simulink model "LQR_Simulation"  (R2022b)
settings: Solver=ode45  StartTime=0.0  StopTime=inf  RelTol=1e-3
values from neighbouring files (symbols this model uses):
  D = 3    [tunningLQR.m]
  xRef = xRef2s    [tunningLQR.m]
  yRef = yRef2s    [tunningLQR.m]
undefined symbols (not defined in the file or in its folder): curvature, esc, hz, path, Q, R_, velocity
libraries: vehdynlibviscommon x1, dspstat3 x1, autolibshared x1
settings Model: Creator=kisho  LastModifiedBy=kisho
settings OptimizationCC: DefaultParameterBehavior=Inlined  EnhancedBackFolding=on  PassReuseOutputArgsAs=Individual arguments  ZeroExternalMemoryAtStartup=off  ZeroInternalMemoryAtStartup=off  MaxStackSize=64  OptimizeBlockOrder=speed  DifferentSizesBufferReuse=on  OptimizationCustomize=off  EfficientTunableParamExpr=on
settings DebuggingCC: ParameterTunabilityLossMsg=error  UnconnectedInputMsg=warning  UnconnectedOutputMsg=warning  UnconnectedLineMsg=warning
settings HardwareCC: ProdBitPerPointer=32  ProdBitPerSizeT=32  ProdBitPerPtrDiffT=32  ProdLargestAtomicFloat=None  ProdIntDivRoundTo=Undefined  ProdEndianess=Unspecified  ProdWordSize=32  ProdHWDeviceType=ASIC/FPGA->ASIC/FPGA  TargetBitPerPointer=64  TargetBitPerSizeT=64  TargetBitPerPtrDiffT=64  TargetLongLongMode=on  TargetIntDivRoundTo=Zero  TargetEndianess=LittleEndian  TargetWordSize=64  TargetHWDeviceType=Custom Processor->MATLAB Host Computer  ProdEqTarget=off
settings ModelReferenceCC: EnableRefExpFcnMdlSchedulingChecks=on
settings SFSimCC: MATLABDynamicMemAlloc=off
settings RTWCC: Description=Embedded Coder  SystemTargetFile=ert.tlc  TemplateMakefile=ert_default_tmf  Toolchain=Catkin  DLArmComputeVersion=19.05
settings CodeAppCC: ForceParamTrailComments=on  IgnoreCustomStorageClasses=off  OperatorAnnotations=on  SimulinkDataObjDesc=on  SFDataObjDesc=on  InsertBlockDesc=on
settings ERTTargetCC: InlinedParameterPlacement=NonHierarchical  ERTCustomFileTemplate=example_file_process.tlc

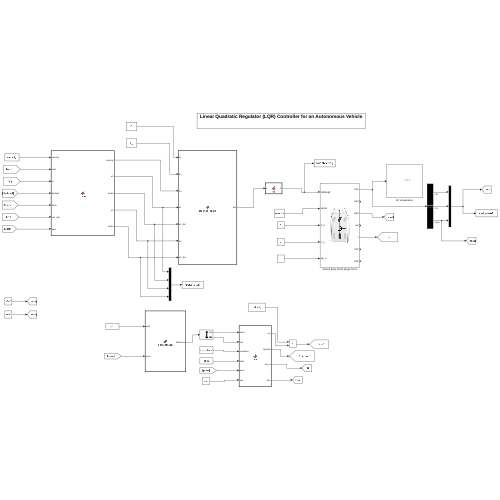
[thumbnail: Simulink's stored preview of the top-level diagram]
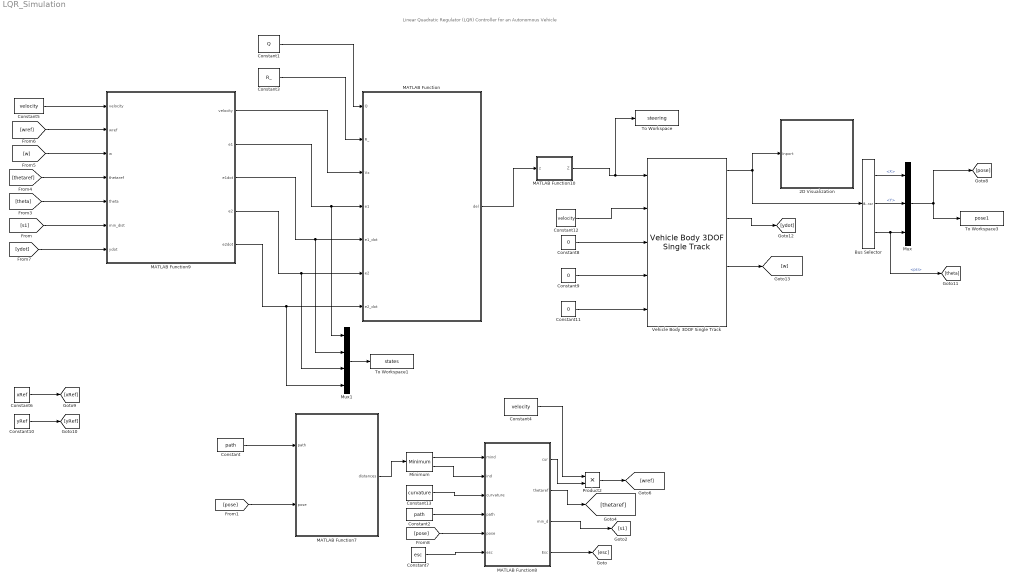
== system LQR_Simulation ==
  note: Linear Quadratic Regulator (LQR) Controller for an Autonomous Vehicle
  2D Visualization : Subsystem
      mask Display: image("visualization.JPG");
  Bus Selector : BusSelector  OutputSignals=InertFrm.Cg.Disp.X,InertFrm.Cg.Disp.Y,InertFrm.Cg.Ang.psi
  Constant : Constant  Value=path  SampleTime=1/hz
  Constant1 : Constant  Value=Q  SampleTime=1/hz
  Constant10 : Constant  Value=yRef  SampleTime=1/hz
  Constant11 : Constant  Value=0  SampleTime=1/hz
  Constant12 : Constant  Value=velocity  SampleTime=1/hz
  Constant13 : Constant  Value=curvature  SampleTime=1/hz
  Constant2 : Constant  Value=path  SampleTime=1/hz
  Constant3 : Constant  Value=R_  SampleTime=1/hz
  Constant4 : Constant  Value=velocity  SampleTime=1/hz
  Constant5 : Constant  Value=velocity  SampleTime=1/hz
  Constant6 : Constant  Value=xRef  SampleTime=1/hz
  Constant7 : Constant  Value=esc  SampleTime=1/hz
  Constant8 : Constant  Value=0  SampleTime=1/hz
  Constant9 : Constant  Value=0  SampleTime=1/hz
  MATLAB Function : MATLAB Function  TreatAsAtomicUnit=on
  MATLAB Function10 : MATLAB Function  TreatAsAtomicUnit=on
  MATLAB Function7 : MATLAB Function  TreatAsAtomicUnit=on
  MATLAB Function8 : MATLAB Function  TreatAsAtomicUnit=on
  MATLAB Function9 : MATLAB Function  TreatAsAtomicUnit=on
  Minimum : dspstat3/Minimum  operation=minimum  fcn=Value and Index  indexBase=One  operateOver=Each row  Dimension=1  InputProcessing=Columns as channels (frame based)  reset=None  roiEnable=off  roiType=Rectangles  roiPortion=Entire ROI  roiOutput=Individual statistics for each ROI  roiFlag=off  roundingMode=Floor  overflowMode=off
  Mux : Mux  Inputs=3
  Mux1 : Mux
  Product2 : Product
  To Workspace : ToWorkspace  VariableName=steering  SaveFormat=Structure With Time  SampleTime=-1
  To Workspace1 : ToWorkspace  VariableName=states  SaveFormat=Structure With Time  SampleTime=-1
  To Workspace3 : ToWorkspace  VariableName=pose1  SaveFormat=Structure With Time  SampleTime=-1
  Vehicle Body 3DOF Single Track : autolibshared/Vehicle Body 3DOF Single Track  trackMode=Single (bicycle)  inputMode=External longitudinal velocity  frontSteerMode=on  rearSteerMode=off  windMode=off  muMode=off  extFMode=off  extMMode=off  htchFMode=off  htchMMode=off  extXo=on  extpsio=on  extxdoto=off  extro=off  extYo=on  extTamb=off  extydoto=off  aMode=2  NF=2  NR=2  m=5  a=0.15  b=0.15  h=0  dh=1  hh=0.2  X_o=0  xdot_o=0  CalphaMode=off  sigmaMode=on  d=0  hl=0  w=[1.4,1.4]  Cy_f=12e3  Cy_r=11e3  sigma_f=.1  sigma_r=.1  alpha_f_brk=[-.1 .1]  Cy_f_data=[-9e3 9e3]  alpha_r_brk=[-.1 .1]  Cy_r_data=[-9e3 9e3]  Y_o=0  ydot_o=0  Izz=0.05  psi_o=0  r_o=0  Af=2  Cd=.3  Cl=.1  Cpm=.1  beta_w=[0 0.01:0.01:0.3]  Cs=[0 0.01:0.01:0.3]  Cym=[0 1e-6:0.01:0.3]  Pabs=101325  Tair=273  g=9.81  mu=1  xdot_tol=.01  Fznom=5000  Fxtire_sat=7e4  Fytire_sat=7e4  longOff=0  latOff=0  vertOff=0  wrapAng=off
  wires:
  MATLAB Function/1(del) -> MATLAB Function10/1(z)
  [s1] -> MATLAB Function9/6(min_dist)
  [theta] -> MATLAB Function9/5(theta)
  [thetaref] -> MATLAB Function9/4(thetaref)
  [w] -> MATLAB Function9/3(w)
  [wref] -> MATLAB Function9/2(wref)
  Constant5/1 -> MATLAB Function9/1("velocity ")
  [ydot] -> MATLAB Function9/7(ydot)
  MATLAB Function9/4(e2) -> Mux1/3, MATLAB Function/6(e2)
  MATLAB Function9/1(velocity) -> MATLAB Function/3(Vx)
  Constant3/1 -> MATLAB Function/2(R_)
  Constant1/1 -> MATLAB Function/1(Q)
  Bus Selector/1 -> Mux/1  "<X>"
  Bus Selector/3 -> [theta], Mux/3  "<psi>"
  Vehicle Body 3DOF Single Track/1 -> Bus Selector/1, 2D Visualization/1(Inport)
  Mux/1 -> To Workspace3/1, [pose]
  Bus Selector/2 -> Mux/2  "<Y>"
  Constant9/1 -> Vehicle Body 3DOF Single Track/4
  Constant8/1 -> Vehicle Body 3DOF Single Track/3
  Constant11/1 -> Vehicle Body 3DOF Single Track/5
  Constant12/1 -> Vehicle Body 3DOF Single Track/2
  MATLAB Function10/1(Z) -> To Workspace/1, Vehicle Body 3DOF Single Track/1
  Vehicle Body 3DOF Single Track/3 -> [ydot]
  Constant6/1 -> [xRef]
  Constant10/1 -> [yRef]
  MATLAB Function8/1(cur) -> Product2/2
  Constant7/1 -> MATLAB Function8/6(esc)
  MATLAB Function8/3(min_d) -> [s1]
  MATLAB Function8/4(Esc) -> [esc]
  Constant4/1 -> Product2/1
  Minimum/1 -> MATLAB Function8/1(mind)
  Constant/1 -> MATLAB Function7/1(path)
  Constant2/1 -> MATLAB Function8/4(path)
  Minimum/2 -> MATLAB Function8/2(ind)
  Product2/1 -> [wref]
  [pose] -> MATLAB Function8/5(pose)
  MATLAB Function8/2(thetaref) -> [thetaref]
  MATLAB Function7/1(distances) -> Minimum/1
  Constant13/1 -> MATLAB Function8/3(curvature)
  [pose] -> MATLAB Function7/2(pose)
  Vehicle Body 3DOF Single Track/5 -> [w]
  MATLAB Function9/2(e1) -> Mux1/1, MATLAB Function/4(e1)
  Mux1/1 -> To Workspace1/1
  MATLAB Function9/3(e1dot) -> Mux1/2, MATLAB Function/5(e1_dot)
  MATLAB Function9/5(e2dot) -> Mux1/4, MATLAB Function/7(e2_dot)

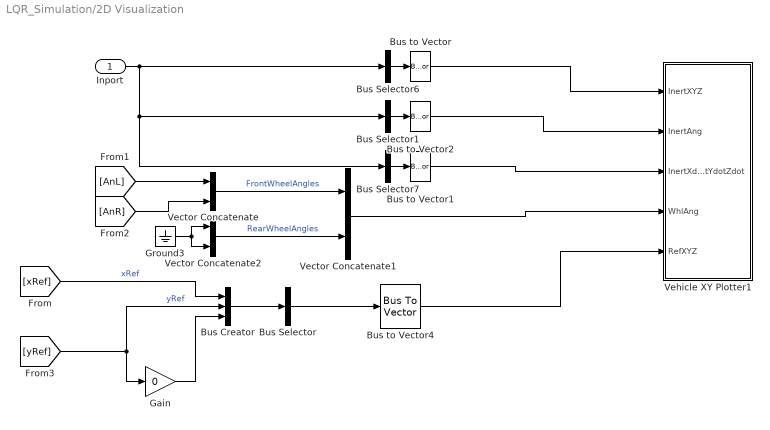
== system LQR_Simulation/2D Visualization ==
  Inport : Inport
  Bus Creator : BusCreator  Inputs=3
  Bus Selector : BusSelector  OutputSignals=xRef,yRef,signal3  OutputAsBus=on
  Bus Selector1 : BusSelector  OutputSignals=InertFrm.Cg.Ang.phi,InertFrm.Cg.Ang.theta,InertFrm.Cg.Ang.psi  OutputAsBus=on
  Bus Selector6 : BusSelector  OutputSignals=InertFrm.Geom.Disp.X,InertFrm.Geom.Disp.Y,InertFrm.Geom.Disp.Z  OutputAsBus=on
  Bus Selector7 : BusSelector  OutputSignals=InertFrm.Geom.Vel.Xdot,InertFrm.Geom.Vel.Ydot,InertFrm.Geom.Vel.Zdot  OutputAsBus=on
  Bus to Vector{,1..2,4} (4 alike) : BusToVector
  Gain : Gain  Gain=0
  Ground3 : Ground
  Vector Concatenate : Concatenate
  Vector Concatenate1 : Concatenate
  Vector Concatenate2 : Concatenate
  Vehicle XY Plotter1 : Subsystem  mask(Vehicle XY Plotter){extRef=on, extStats=off, extTireF=off, a=2, b=2, w=2, figBorder=10, bufferSize=1024, velNorm=5, tireFNorm=1000, pltDT=0.2}
      mask prompts: extRef "Plot path reference, extRef"; extStats "Display speed, RPM and Gear"; extTireF "Display tire forces"; a "Distance to front axle from CG, a [m]:"; b "Distance to rear axle from CG, b [m]:"; w "Track width, w [m]:"; figBorder "Distance to figure borders, figBorder [m]:"; bufferSize "Path buffer sampe size, bufferSize []:"; velNorm "Velocity vector scaling, velNorm [m*s/m]:"; tireFNorm "Tire force vector scaling, tireFNorm [m/N]:"; pltDT "Plot update rate, pltDT [s]:"
      mask help:
      | This block will display a MATLAB figure which indicates the vehicle path, current position and heading velocity.
      | An optional path reference is also provided.
      mask init:
      | block = gcb;
      | if autoblkschecksimstopped(block)
      |     ParamNames = {'extRef';'extStats';'extTireF';'extTireF'};
      |     PortNames = {'RefXYZ';'Stats';'TireFx';'TireFy'};
      |     for idx=1:length(PortNames)
      |         InportOption  = {'built-in/Ground', [PortNames{idx}, ' Ground'];...
      |             'built-in/Inport',PortNames{idx}};
      |         if ~strcmp(get_param(block,ParamNames{idx}),'on')
      |             NewBlkHdl = autoblksreplaceblock(block, InportOption, 1);
      |             set_param(NewBlkHdl, 'ShowName', 'off');
      |         else
      |             autoblksreplaceblock(block, InportOption, 2);
      |         end
      |     end
      |     InportNames = {'InertXYZ';'InertAng';'InertXdotYdotZdot';'WhlAng';'RefXYZ';'Stats';'TireFx';'TireFy'};
      |     FoundNames = get_param(find_system(block, 'LookUnderMasks', 'all', 'SearchDepth', 1, 'FollowLinks', 'on', 'BlockType', 'Inport'), 'Name');
      |     [~,PortI] = intersect(InportNames, FoundNames);
      |     PortI = sort(PortI);
      |     for idx = 1:length(PortI)
      |         set_param([block, '/', InportNames{PortI(idx)}], 'Port', num2str(idx));
      |     end
      | end
      mask TypeOptions a: Vehicle XY Plotter/a
      mask TypeOptions b: Vehicle XY Plotter/b
      mask TypeOptions w: Vehicle XY Plotter/w
      mask TypeOptions figBorder: Vehicle XY Plotter/figBorder
      mask TypeOptions bufferSize: Vehicle XY Plotter/bufferSize
      mask TypeOptions velNorm: Vehicle XY Plotter/velNorm
      mask TypeOptions tireFNorm: Vehicle XY Plotter/tireFNorm
      mask DialogControl Container3 Prompt: Plot and Display Options
  wires:
  Bus Creator/1 -> Bus Selector/1
  [xRef] -> Bus Creator/1  "xRef"
  Gain/1 -> Bus Creator/3
  [yRef] -> Gain/1, Bus Creator/2  "yRef"
  Bus Selector/1 -> Bus to Vector4/1
  Bus to Vector4/1 -> Vehicle XY Plotter1/5(RefXYZ)
  Inport/1 -> Bus Selector6/1, Bus Selector1/1, Bus Selector7/1
  [AnR] -> Vector Concatenate/2
  Bus Selector1/1 -> Bus to Vector2/1
  Bus to Vector2/1 -> Vehicle XY Plotter1/2(InertAng)
  Bus to Vector/1 -> Vehicle XY Plotter1/1(InertXYZ)
  Bus to Vector1/1 -> Vehicle XY Plotter1/3(InertXdotYdotZdot)
  Bus Selector7/1 -> Bus to Vector1/1
  Vector Concatenate2/1 -> Vector Concatenate1/2  "RearWheelAngles"
  [AnL] -> Vector Concatenate/1
  Vector Concatenate/1 -> Vector Concatenate1/1  "FrontWheelAngles"
  Bus Selector6/1 -> Bus to Vector/1
  Ground3/1 -> Vector Concatenate2/2, Vector Concatenate2/1
  Vector Concatenate1/1 -> Vehicle XY Plotter1/4(WhlAng)

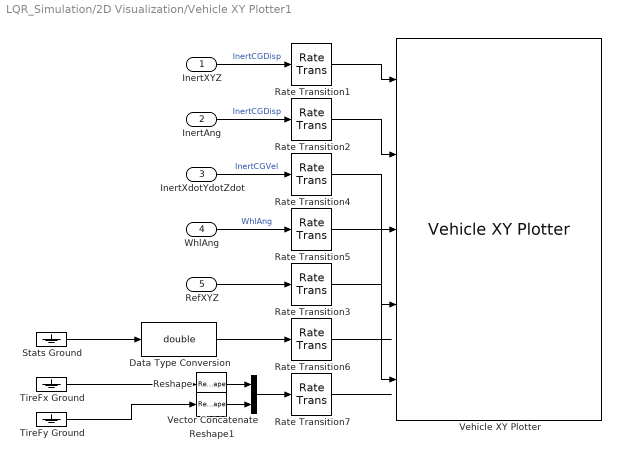
== system LQR_Simulation/2D Visualization/Vehicle XY Plotter1 ==
  InertXYZ : Inport
  InertAng : Inport  Port=2
  InertXdotYdotZdot : Inport  Port=3
  WhlAng : Inport  Port=4
  RefXYZ : Inport  Port=5
  Data Type Conversion : DataTypeConversion  OutDataTypeStr=double  SaturateOnIntegerOverflow=off  RndMeth=Floor
  Rate Transition{1..7} (7 alike) : RateTransition  Deterministic=off  OutPortSampleTime=pltDT
  Reshape : Reshape  OutputDimensionality=Row vector (2-D)
  Reshape1 : Reshape  OutputDimensionality=Row vector (2-D)
  Stats Ground : Ground
  TireFx Ground : Ground
  TireFy Ground : Ground
  Vector Concatenate : Concatenate  Mode=Multidimensional array
  Vehicle XY Plotter : vehdynlibviscommon/Vehicle XY Plotter  w=w  a=a  b=b  figBorder=figBorder  bufferSize=bufferSize  extStats=off  extTireF=off
  wires:
  TireFy Ground/1 -> Reshape1/1
  TireFx Ground/1 -> Reshape/1
  Stats Ground/1 -> Data Type Conversion/1
  InertAng/1 -> Rate Transition2/1  "InertCGDisp"
  InertXdotYdotZdot/1 -> Rate Transition4/1  "InertCGVel"
  InertXYZ/1 -> Rate Transition1/1  "InertCGDisp"
  WhlAng/1 -> Rate Transition5/1  "WhlAng"
  Rate Transition3/1 -> Vehicle XY Plotter/5
  Rate Transition1/1 -> Vehicle XY Plotter/1
  Rate Transition2/1 -> Vehicle XY Plotter/2
  Rate Transition4/1 -> Vehicle XY Plotter/3
  Rate Transition5/1 -> Vehicle XY Plotter/4
  Rate Transition6/1 -> ?
  Data Type Conversion/1 -> Rate Transition6/1
  Rate Transition7/1 -> ?
  RefXYZ/1 -> Rate Transition3/1
  Reshape/1 -> Vector Concatenate/1
  Reshape1/1 -> Vector Concatenate/2
  Vector Concatenate/1 -> Rate Transition7/1

== matlab function LQR_Simulation/MATLAB Function ==
  data: Q input; R_ input; del output; Vx input; e1 input; e1_dot input; e2 input; e2_dot input
function del = steering_angle(Q,R_,Vx,e1,e1_dot, e2, e2_dot)

% defining vehicle parameters
a = 0.330/2;     % m ,distance from CoG to front axel
b = 0.330/2;     % m ,distance from CoG to rear axel
Iz = 5*0.1^2;  % kg-m^2 ,Yaw rate of inertia around CoG
m = 5;     % kg ,mass of the vehicle 
Cf = 8354;   % N/rad ,cornering stiffness of the front axel
Cr = 8310;   % N/rad ,cornering stiffness of the rear axel
w = 0.25 ;   % m ,vehicle width
lf = 0.330/2;    % m ,CoG to front end 
lr = 0.330/2;    % m ,CoG to rear end

% state space and control inpute's coefficient matrix
A = [0,1,0,0;
    0,-(2*Cf+2*Cr)/(m*Vx),(2*Cf+2*Cf)/(m),(-2*Cf*lf+2*Cf*lr)/(m*Vx);
    0,0,0,1;
    0,-(2*Cf*lf-2*Cf*lr)/(Iz*Vx),(2*Cf*lf-2*Cf*lr)/(Iz),-(2*Cf*lf^2+2*Cf*lr^2)/(Iz*Vx)];

B1 = [0; ((-2*Cf+Cf)/(m*Vx)-Vx); 0; -(2*Cf*lf^2+2*Cf*lr^2)/(Iz*Vx)];

B = [0; (2*Cf/m); 0; (2*Cf*lf/Iz)];

B2 = [0;0;0;1];
%Q = diag([5 0 5 1]);
%R = 10;

% calculating gain matrix
K = lqr_own(A, B, Q, R_);

% state space matrix
X = [e1;e1_dot; e2; e2_dot];



del = [-K*X];

== matlab function LQR_Simulation/MATLAB Function7 ==
  data: path input; distances output; pose input
function distances  = nearestPose(path, pose)
    % path: Nx3 matrix containing the x, y, and heading of the waypoints in the path
    % current_pose: 1x3 vector containing the x, y, and heading of the current pose of the vehicle
    % nearest_pose: 1x3 vector containing the x, y, and heading of the nearest pose on the path
    % nearest_index: index of the nearest pose on the path
    
    % Find the distance from the current pose to each waypoint on the path
    
    l = length(path(:,1));
    cx = path(:,1);
    cy = path(:,2);
    dx = zeros(l);
    dy = zeros(l);
    distances =  zeros(1,l);


    for i = 1:l
        dx(i) = pose(1) - cx(i);
        dy(i) = pose(2) - cy(i);
        distances(i) = sqrt((dx(i)^2+dy(i)^2));
    end
end

== matlab function LQR_Simulation/MATLAB Function8 ==
  data: mind input; ind input; curvature input; cur output; path input; thetaref output; pose input; min_d output; esc input; Esc output
function [cur,thetaref,min_d,Esc] = fcn(mind,ind,curvature,path,pose,esc)

cur = curvature(ind);
thetaref = path(ind,3);

% cross track error

current_position = [pose(1);pose(2)];
next_waypoint = [path(ind+1,1);path(ind+1,2)];

waypoint_vector = next_waypoint - current_position;
normal_vector = [-waypoint_vector(2), waypoint_vector(1)];
vehicle_heading = [cos(pose(3)), sin(pose(3))];
dot_product = dot(vehicle_heading, normal_vector);
if dot_product > 0
    cross_track_error = +1; % vehicle is to the right of the line
else
    cross_track_error = -1; % vehicle is to the left of the line
end
min_d = mind*cross_track_error;


%%% stopping the vehicle when vehicle reaching near the target point

if (ind >= length(path)-2)
    Esc = 0;
else
    Esc = esc;
end

end

== matlab function LQR_Simulation/MATLAB Function9 ==
  data: velocity output; velocity input; wref input; e1 output; e1dot output; e2 output; e2dot output; w input; thetaref input; theta input; min_dist input; ydot input
function [velocity,e1,e1dot,e2,e2dot]= state(velocity,wref,w,thetaref,theta,min_dist,ydot)

% rate change of heading error
 e2dot = w - wref;

% heading error 
 e2    = theta -thetaref;
if e2 <= -pi
    e2 = theta + (pi-thetaref);
elseif e2 >= pi
    e2 = -(pi-theta+thetaref);
end

% cross track error
 e1 = min_dist;
 e1dot = ydot+velocity*(e2);


end

== matlab function LQR_Simulation/MATLAB Function10 ==
  data: z input; Z output
function Z = fcn(z)

if (z > pi/6)
    z = pi/6;
elseif (z < -pi/6)
    z = -pi/6;
else
    z =z;
end

Z = z;
end
